simulink model "oob_detector"  (R2018a)
settings: Solver=VariableStepAuto  StartTime=0.0  StopTime=100  FixedStep=0.01  RelTol=1e-3
settings Model: Creator=blond  LastModifiedBy=blond

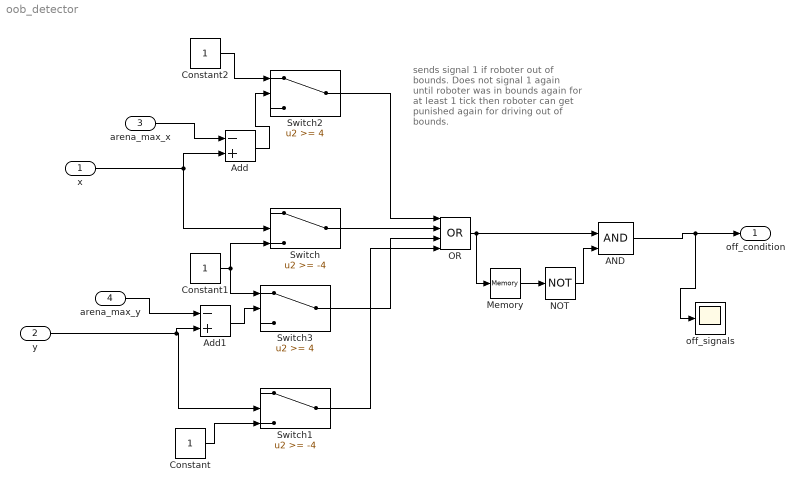
== system oob_detector ==
  note: sends signal 1 if roboter
      | out of bounds. Does not
      | signal 1 again until
      | roboter was in bounds
      | again for at least 1 tick
      | then roboter can get
      | punished again for
      | driving out of bounds.
  x : Inport
  y : Inport  Port=2
  "arena_max_x " : Inport  Port=3
  arena_max_y : Inport  Port=4
  AND : Logic  IconShape=distinctive  AllPortsSameDT=off  OutDataTypeStr=boolean
  Add : Sum  Inputs=-+
  Add1 : Sum  Inputs=-+
  Constant : Constant
  Constant1 : Constant
  Constant2 : Constant
  Memory : Memory
  NOT : Logic  Operator=NOT  IconShape=distinctive  AllPortsSameDT=off  OutDataTypeStr=boolean
  OR : Logic  Operator=OR  Inputs=4  IconShape=distinctive  AllPortsSameDT=off  OutDataTypeStr=boolean
  Switch : Switch  Threshold=-4
  Switch1 : Switch  Threshold=-4
  Switch2 : Switch  Threshold=4
  Switch3 : Switch  Threshold=4
  off_signals : Scope
  off_condition : Outport
  wires:
  x/1 -> Add/2, Switch/2
  y/1 -> Add1/2, Switch1/2
  Constant/1 -> Switch1/3
  Constant1/1 -> Switch/3, Switch3/1
  Constant2/1 -> Switch2/1
  Switch2/1 -> OR/1
  Switch/1 -> OR/2
  Switch3/1 -> OR/3
  Switch1/1 -> OR/4
  OR/1 -> Memory/1, AND/1
  Memory/1 -> NOT/1
  NOT/1 -> AND/2
  AND/1 -> off_signals/1, off_condition/1
  "arena_max_x "/1 -> Add/1
  Add/1 -> Switch2/2
  Add1/1 -> Switch3/2
  arena_max_y/1 -> Add1/1
